simulink model "Modelo_nolineal_5GDL_EMS_2022"  (R2021b)
settings: Solver=VariableStepAuto  StartTime=0.0  StopTime=5  FixedStep=T  RelTol=1e-3
undefined symbols (not defined in the file or in its folder): AG0, l1, l2, l3, pod, ROTZ_0, y_ini
settings Model: Creator=EDMAOR  LastModifiedBy=emate
settings SolverCC: AlgebraicLoopSolver=TrustRegion
settings DebuggingCC: SFMachineParentedDataDiag=warning
settings SFSimCC: CustomCodeUndefinedFunction=UseInterfaceOnly

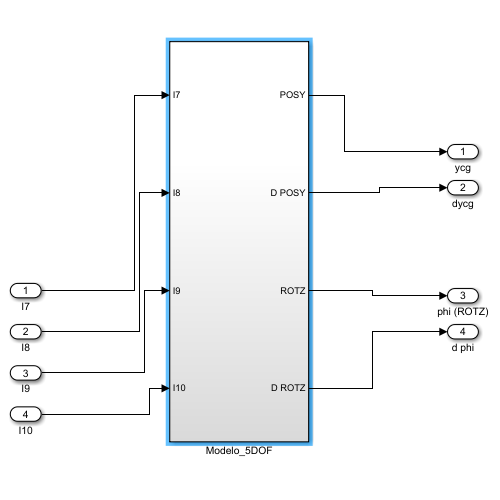
[thumbnail: Simulink's stored preview of the top-level diagram]
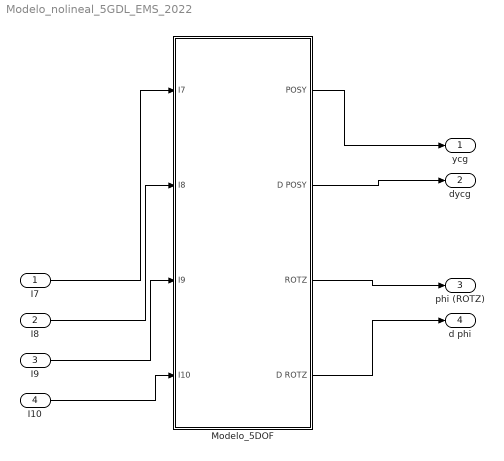
== system Modelo_nolineal_5GDL_EMS_2022 ==
  I7 : Inport
  I8 : Inport  Port=2
  I9 : Inport  Port=3
  I10 : Inport  Port=4
  Modelo_5DOF : Subsystem
  ycg : Outport  VectorParamsAs1DForOutWhenUnconnected=off
  dycg : Outport  Port=2  VectorParamsAs1DForOutWhenUnconnected=off
  phi (ROTZ) : Outport  Port=3  VectorParamsAs1DForOutWhenUnconnected=off
  d phi : Outport  Port=4  VectorParamsAs1DForOutWhenUnconnected=off
  wires:
  Modelo_5DOF/1(POSY) -> ycg/1
  Modelo_5DOF/2(D POSY) -> dycg/1
  Modelo_5DOF/3(ROTZ) -> phi (ROTZ)/1
  Modelo_5DOF/4(D ROTZ) -> d phi/1
  I7/1 -> Modelo_5DOF/1(I7)
  I8/1 -> Modelo_5DOF/2(I8)
  I9/1 -> Modelo_5DOF/3(I9)
  I10/1 -> Modelo_5DOF/4(I10)

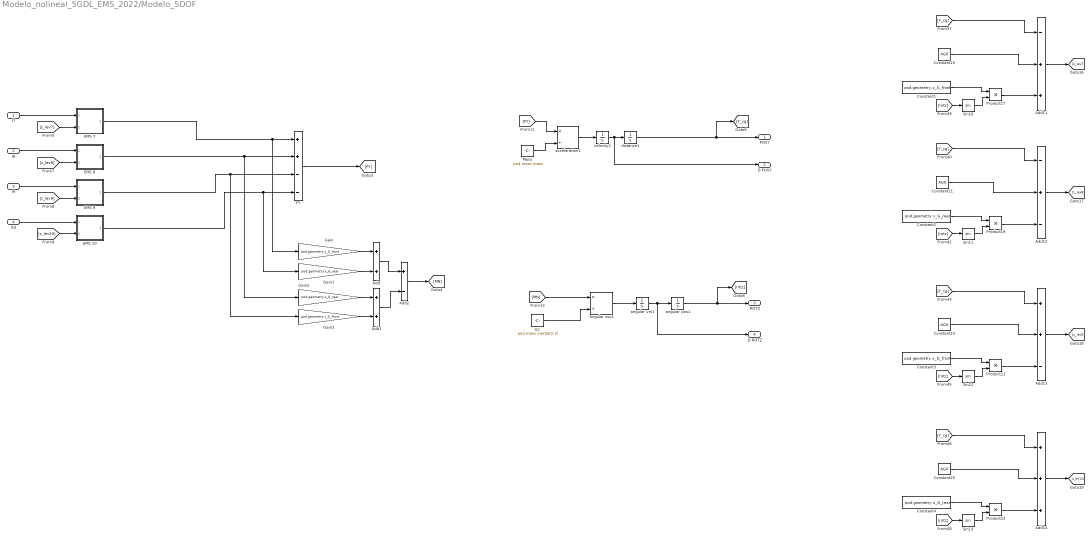
== system Modelo_nolineal_5GDL_EMS_2022/Modelo_5DOF ==
  I7 : Inport
  I8 : Inport  Port=2
  I9 : Inport  Port=3
  I10 : Inport  Port=4
  Add : Sum
  Add1 : Sum
  Add11 : Sum  Inputs=-++
  Add12 : Sum  Inputs=-+-
  Add13 : Sum  Inputs=++-
  Add14 : Sum  Inputs=+++
  Add2 : Sum  Inputs=+-
  Constant1 : Constant  Value=pod.geometry.x_G_front
  Constant{19,21,23,25} (4 alike) : Constant  Value=AG0
  Constant2 : Constant  Value=pod.geometry.x_G_rear
  Constant3 : Constant  Value=pod.geometry.x_G_front
  Constant4 : Constant  Value=pod.geometry.x_G_rear
  EMS 10 : Subsystem
  EMS 7 : Subsystem
  EMS 8 : Subsystem
  EMS 9 : Subsystem
  FY : Sum  Inputs=++--
  Gain : Gain  Gain=pod.geometry.x_G_front
  Gain1 : Gain  Gain=pod.geometry.x_G_rear
  Gain2 : Gain  Gain=pod.geometry.x_G_rear
  Gain3 : Gain  Gain=pod.geometry.x_G_front
  Izz : Constant  Value=pod.mass.inertia(3,3)
  Mass : Constant  Value=pod.mass.mass
  Product{17,19,21,23} (4 alike) : Product
  Sin{10..13} (4 alike) : Trigonometry
  acceleration1 : Product  Inputs=*/
  angular acc1 : Product  Inputs=*/
  angular pos1 : Integrator  InitialCondition=ROTZ_0
  angular vel1 : Integrator
  distance1 : Integrator  InitialCondition=y_ini
  velocity1 : Integrator
  POSY : Outport  VectorParamsAs1DForOutWhenUnconnected=off
  D POSY : Outport  Port=2  VectorParamsAs1DForOutWhenUnconnected=off
  ROTZ : Outport  Port=3  VectorParamsAs1DForOutWhenUnconnected=off
  D ROTZ : Outport  Port=4  VectorParamsAs1DForOutWhenUnconnected=off
  wires:
  I7/1 -> EMS 7/1(current 7)
  [z_lev7] -> EMS 7/2(distance 7)
  I8/1 -> EMS 8/1(current 8)
  [z_lev8] -> EMS 8/2(distance 8)
  I9/1 -> EMS 9/1(current 9)
  [z_lev9] -> EMS 9/2(distance 9)
  I10/1 -> EMS 10/1(current 10)
  [z_lev10] -> EMS 10/2(distance 10)
  EMS 7/1(EMS 7) -> Gain/1, FY/1
  EMS 8/1(EMS 8) -> Gain2/1, FY/2
  EMS 9/1(EMS 9) -> Gain3/1, FY/3
  EMS 10/1(EMS 10) -> Gain1/1, FY/4
  FY/1 -> [FY]
  [FY] -> acceleration1/1
  Mass/1 -> acceleration1/2
  distance1/1 -> [Y_cg], POSY/1
  velocity1/1 -> distance1/1, D POSY/1
  acceleration1/1 -> velocity1/1
  angular acc1/1 -> angular vel1/1
  Izz/1 -> angular acc1/2
  angular vel1/1 -> D ROTZ/1, angular pos1/1
  [MN] -> angular acc1/1
  angular pos1/1 -> [rotz], ROTZ/1
  Add11/1 -> [z_lev7]
  Product17/1 -> Add11/3
  Constant1/1 -> Product17/1
  Sin10/1 -> Product17/2
  [rotz] -> Sin10/1
  Constant19/1 -> Add11/2
  [Y_cg] -> Add11/1
  [Y_cg] -> Add12/1
  Constant21/1 -> Add12/2
  [rotz] -> Sin11/1
  Sin11/1 -> Product19/2
  Constant2/1 -> Product19/1
  Product19/1 -> Add12/3
  Add12/1 -> [z_lev8]
  Add13/1 -> [z_lev9]
  Product21/1 -> Add13/3
  Constant3/1 -> Product21/1
  Sin12/1 -> Product21/2
  [rotz] -> Sin12/1
  Constant23/1 -> Add13/2
  Constant25/1 -> Add14/2
  [rotz] -> Sin13/1
  Sin13/1 -> Product23/2
  Constant4/1 -> Product23/1
  Product23/1 -> Add14/3
  Add14/1 -> [z_lev10]
  [Y_cg] -> Add13/1
  [Y_cg] -> Add14/1
  Gain/1 -> Add/1
  Gain1/1 -> Add/2
  Gain2/1 -> Add1/1
  Gain3/1 -> Add1/2
  Add2/1 -> [MN]
  Add/1 -> Add2/1
  Add1/1 -> Add2/2

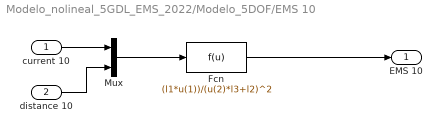
== system Modelo_nolineal_5GDL_EMS_2022/Modelo_5DOF/EMS 10 ==
  current 10 : Inport
  distance 10 : Inport  Port=2
  Fcn : Fcn  Expr=(l1*u(1))/(u(2)*l3+l2)^2
  Mux : Mux  Inputs=2
  EMS 10 : Outport  VectorParamsAs1DForOutWhenUnconnected=off
  wires:
  Fcn/1 -> EMS 10/1
  Mux/1 -> Fcn/1
  distance 10/1 -> Mux/2
  current 10/1 -> Mux/1

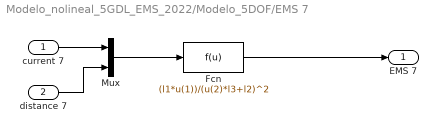
== system Modelo_nolineal_5GDL_EMS_2022/Modelo_5DOF/EMS 7 ==
  current 7 : Inport
  distance 7 : Inport  Port=2
  Fcn : Fcn  Expr=(l1*u(1))/(u(2)*l3+l2)^2
  Mux : Mux  Inputs=2
  EMS 7 : Outport  VectorParamsAs1DForOutWhenUnconnected=off
  wires:
  current 7/1 -> Mux/1
  distance 7/1 -> Mux/2
  Mux/1 -> Fcn/1
  Fcn/1 -> EMS 7/1

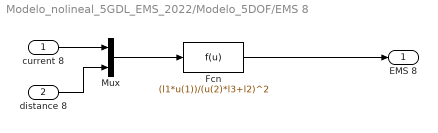
== system Modelo_nolineal_5GDL_EMS_2022/Modelo_5DOF/EMS 8 ==
  current 8 : Inport
  distance 8 : Inport  Port=2
  Fcn : Fcn  Expr=(l1*u(1))/(u(2)*l3+l2)^2
  Mux : Mux  Inputs=2
  EMS 8 : Outport  VectorParamsAs1DForOutWhenUnconnected=off
  wires:
  Fcn/1 -> EMS 8/1
  Mux/1 -> Fcn/1
  distance 8/1 -> Mux/2
  current 8/1 -> Mux/1

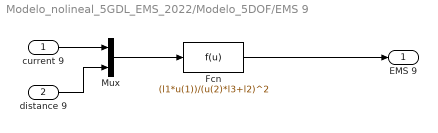
== system Modelo_nolineal_5GDL_EMS_2022/Modelo_5DOF/EMS 9 ==
  current 9 : Inport
  distance 9 : Inport  Port=2
  Fcn : Fcn  Expr=(l1*u(1))/(u(2)*l3+l2)^2
  Mux : Mux  Inputs=2
  EMS 9 : Outport  VectorParamsAs1DForOutWhenUnconnected=off
  wires:
  current 9/1 -> Mux/1
  distance 9/1 -> Mux/2
  Mux/1 -> Fcn/1
  Fcn/1 -> EMS 9/1
